simulink model "FSFB_FF_Controller"  (R2022a)
settings: Solver=VariableStepAuto  StartTime=0.0  StopTime=10.0  RelTol=1e-3
undefined symbols (not defined in the file): K1, K2
libraries: dspsigops x1
settings Model: Creator=domin  LastModifiedBy=domin

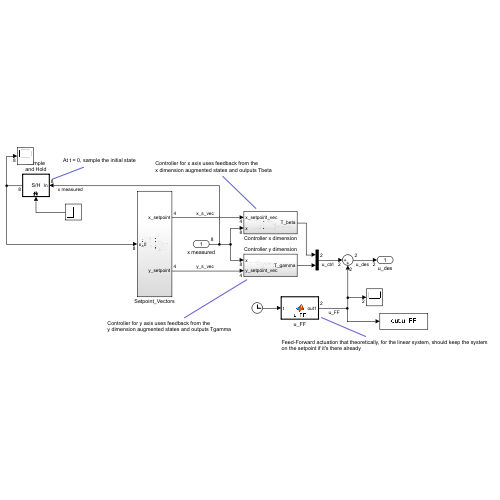
[thumbnail: Simulink's stored preview of the top-level diagram]
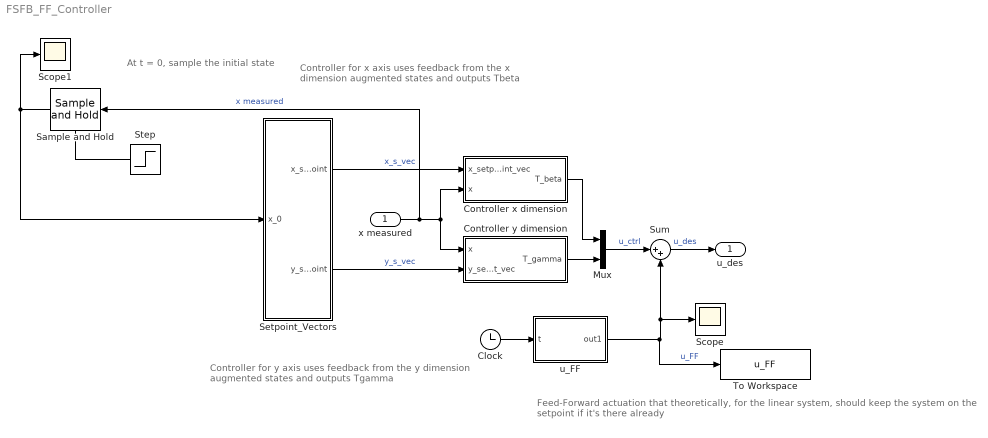
== system FSFB_FF_Controller ==
  note: Controller for x axis uses feedback from the
      | x dimension augmented states and outputs Tbeta
  note: Feed-Forward actuation that theoretically, for the linear system, should keep the system on the setpoint if it's there already
  note: Controller for y axis uses feedback from the
      | y dimension augmented states and outputs Tgamma
  note: At t = 0, sample the initial state
  x measured : Inport
  Clock : Clock
  Controller x dimension : Subsystem
  Controller y dimension : Subsystem
  Mux : Mux  Inputs=2
  Sample and Hold : dspsigops/Sample and Hold  trig=Either edge  initCond=0  latchinput=off
  Scope : Scope
  Scope1 : Scope
  Setpoint_Vectors : Subsystem
  Step : Step  Time=0  SampleTime=0
  Sum : Sum  Inputs=|++
  To Workspace : ToWorkspace  VariableName=u_FF  SampleTime=-1
  u_FF : MATLAB Function  TreatAsAtomicUnit=on
  u_des : Outport
  wires:
  Mux/1 -> Sum/1  "u_ctrl"
  u_FF/1(out1) -> To Workspace/1, Sum/2, Scope/1  "u_FF"
  Setpoint_Vectors/2(y_setpoint) -> Controller y dimension/2(y_setpoint_vec)  "y_s_vec"
  Sum/1 -> u_des/1  "u_des"
  Controller y dimension/1(T_gamma) -> Mux/2
  Clock/1 -> u_FF/1(t)
  Controller x dimension/1(T_beta) -> Mux/1
  Setpoint_Vectors/1(x_setpoint) -> Controller x dimension/1(x_setpoint_vec)  "x_s_vec"
  Sample and Hold/1 -> Setpoint_Vectors/1(x_0), Scope1/1
  Step/1 -> Sample and Hold/Trigger
  x measured/1 -> Sample and Hold/1, Controller y dimension/1(x), Controller x dimension/2(x)  "x measured"

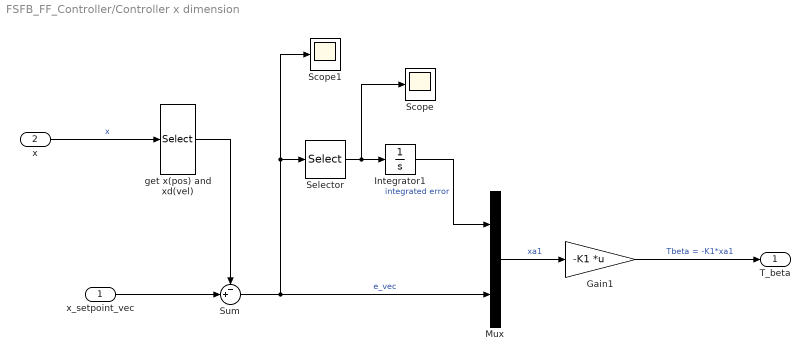
== system FSFB_FF_Controller/Controller x dimension ==
  x_setpoint_vec : Inport
  x : Inport  Port=2
  Gain1 : Gain  Gain=-K1  Multiplication=Matrix(K*u)
  Integrator1 : Integrator
  Mux : Mux  Inputs=2
  Scope : Scope
  Scope1 : Scope
  Selector : Selector  InputPortWidth=4  IndexOptions=Index vector (dialog)  Indices=[1 ]  OutputSizes=1
  Sum : Sum  Inputs=-+|
  get x(pos) and xd(vel) : Selector  InputPortWidth=8  IndexOptions=Index vector (dialog)  Indices=[1:4]  OutputSizes=1
  T_beta : Outport
  wires:
  Gain1/1 -> T_beta/1  "Tbeta = -K1*xa1"
  get x(pos) and xd(vel)/1 -> Sum/1
  Mux/1 -> Gain1/1  "xa1"
  Sum/1 -> Scope1/1, Selector/1, Mux/2  "e_vec"
  x_setpoint_vec/1 -> Sum/2
  x/1 -> get x(pos) and xd(vel)/1  "x"
  Selector/1 -> Scope/1, Integrator1/1
  Integrator1/1 -> Mux/1  "integrated error"

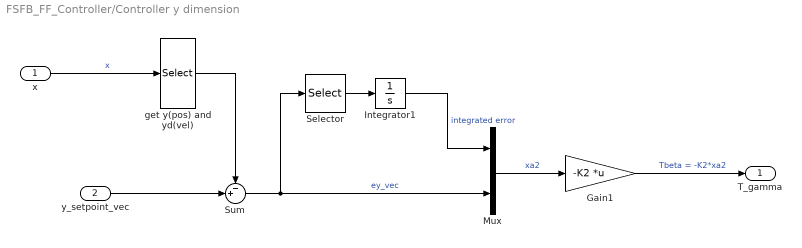
== system FSFB_FF_Controller/Controller y dimension ==
  x : Inport
  y_setpoint_vec : Inport  Port=2
  Gain1 : Gain  Gain=-K2  Multiplication=Matrix(K*u)
  Integrator1 : Integrator
  Mux : Mux  Inputs=2
  Selector : Selector  InputPortWidth=4  IndexOptions=Index vector (dialog)  Indices=[1 ]  OutputSizes=1
  Sum : Sum  Inputs=-+|
  get y(pos) and yd(vel) : Selector  InputPortWidth=8  IndexOptions=Index vector (dialog)  Indices=[5:8]  OutputSizes=1
  T_gamma : Outport
  wires:
  Integrator1/1 -> Mux/1  "integrated error"
  x/1 -> get y(pos) and yd(vel)/1  "x"
  Gain1/1 -> T_gamma/1  "Tbeta = -K2*xa2"
  get y(pos) and yd(vel)/1 -> Sum/1
  Mux/1 -> Gain1/1  "xa2"
  Selector/1 -> Integrator1/1
  Sum/1 -> Selector/1, Mux/2  "ey_vec"
  y_setpoint_vec/1 -> Sum/2

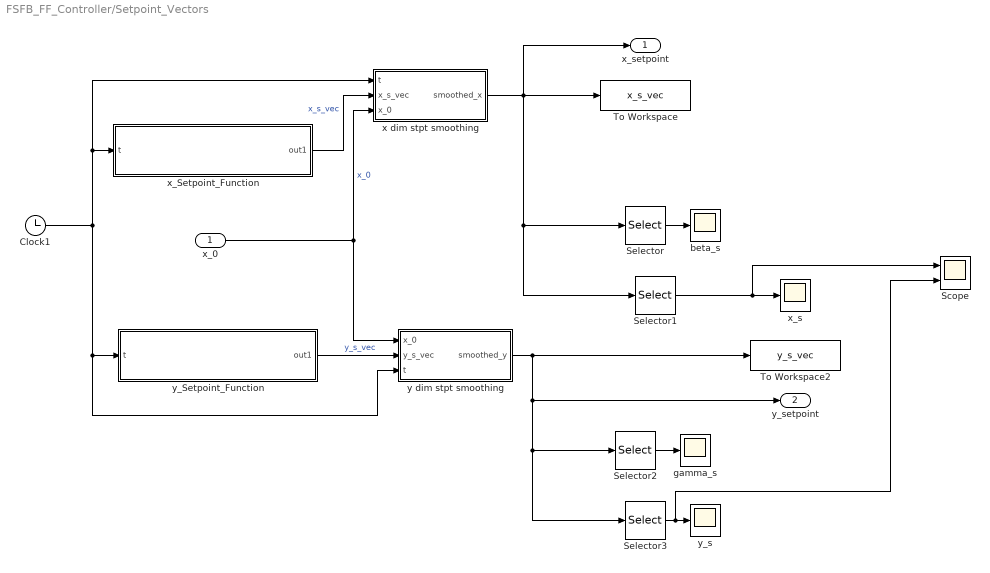
== system FSFB_FF_Controller/Setpoint_Vectors ==
  x_0 : Inport
  Clock1 : Clock
  Scope : Scope  NumInputPorts=2
  Selector : Selector  InputPortWidth=4  IndexOptions=Index vector (dialog)  Indices=[3]  OutputSizes=1
  Selector1 : Selector  InputPortWidth=4  IndexOptions=Index vector (dialog)  Indices=[1]  OutputSizes=1
  Selector2 : Selector  InputPortWidth=4  IndexOptions=Index vector (dialog)  Indices=[3]  OutputSizes=1
  Selector3 : Selector  InputPortWidth=4  IndexOptions=Index vector (dialog)  Indices=[1]  OutputSizes=1
  To Workspace : ToWorkspace  VariableName=x_s_vec  SampleTime=-1
  To Workspace2 : ToWorkspace  VariableName=y_s_vec  SampleTime=-1
  beta_s : Scope
  gamma_s : Scope
  x dim stpt smoothing : MATLAB Function  TreatAsAtomicUnit=on
  x_Setpoint_Function : MATLAB Function  TreatAsAtomicUnit=on
  x_s : Scope
  y dim stpt smoothing : MATLAB Function  TreatAsAtomicUnit=on
  y_Setpoint_Function : MATLAB Function  TreatAsAtomicUnit=on
  y_s : Scope
  x_setpoint : Outport
  y_setpoint : Outport  Port=2
  wires:
  Clock1/1 -> y_Setpoint_Function/1(t), y dim stpt smoothing/3(t), x dim stpt smoothing/1(t), x_Setpoint_Function/1(t)
  x_Setpoint_Function/1(out1) -> x dim stpt smoothing/2(x_s_vec)  "x_s_vec"
  Selector/1 -> beta_s/1
  Selector1/1 -> Scope/1, x_s/1
  Selector3/1 -> Scope/2, y_s/1
  Selector2/1 -> gamma_s/1
  y_Setpoint_Function/1(out1) -> y dim stpt smoothing/2(y_s_vec)  "y_s_vec"
  x dim stpt smoothing/1(smoothed_x) -> Selector/1, Selector1/1, To Workspace/1, x_setpoint/1
  x_0/1 -> y dim stpt smoothing/1(x_0), x dim stpt smoothing/3(x_0)  "x_0"
  y dim stpt smoothing/1(smoothed_y) -> To Workspace2/1, y_setpoint/1, Selector3/1, Selector2/1

== matlab function FSFB_FF_Controller/Setpoint_Vectors/y dim stpt smoothing ==
  data: x_0 input size=8; y_s_vec input; t input; smoothed_y output size=4; Tau parameter
function smoothed_y = fcn(x_0,y_s_vec,t, Tau)

smoothed_y = y_s_vec*(1-exp(-t/Tau)) + x_0(5:end)*exp(-t/Tau);

== matlab function FSFB_FF_Controller/Setpoint_Vectors/x_Setpoint_Function ==
  data: t input; out1 output
function out1 = x_s_vec(t)
%#codegen

%    This function was generated by the Symbolic Math Toolbox version 9.1.
%    08-Jun-2022 13:00:24

t2 = pi.^2;
t3 = t.*pi.*(2.0./5.0);
t4 = t.*pi.*(6.0./5.0);
t5 = cos(t3);
t6 = sin(t3);
t7 = t2.*1.298e+3;
t8 = t7+6.8125e+4;
t9 = t8+5.45e+5;
t10 = 1.0./t8;
t11 = 1.0./t9;
t12 = t10.*5.510882126348228e+4;
t13 = t11.*4.959793913713405e+5;
t14 = t12-5.25e+2./6.49e+2;
t15 = t13-5.25e+2./6.49e+2;
out1 = [t5.*(3.0./4.0e+1)+cos(t4).*(3.0./4.0e+1);t6.*pi.*(-3.0./1.0e+2)-pi.*sin(t4).*(9.0./1.0e+2);-t14.*(t5.*3.0-t5.^3.*4.0)+t5.*t15;t14.*(t6.*pi.*(6.0./5.0)-t5.^2.*t6.*pi.*(2.4e+1./5.0))-t6.*t15.*pi.*(2.0./5.0)];

== matlab function FSFB_FF_Controller/Setpoint_Vectors/y_Setpoint_Function ==
  data: t input; out1 output
function out1 = y_s_vec(t)
%#codegen

%    This function was generated by the Symbolic Math Toolbox version 9.1.
%    08-Jun-2022 13:00:25

t2 = pi.^2;
t3 = pi.^3;
t5 = t.*pi.*(2.0./5.0);
t6 = t.*pi.*(4.0./5.0);
t7 = t.*pi.*(6.0./5.0);
t4 = t2.^2;
t8 = cos(t5);
t9 = cos(t6);
t10 = sin(t5);
t11 = sin(t6);
t13 = t2.*8.842625e+8;
t12 = t4.*1.684804e+6;
t14 = t2.*t9.*1.298e+3;
t15 = t9.*6.13125e+5;
t16 = t12+t13+4.1769140625e+10;
t17 = t14+t15+2.725e+5;
t18 = 1.0./t16;
out1 = [t10.*(-3.0./4.0e+1)+sin(t7).*(3.0./4.0e+1);t8.*pi.*(-3.0./1.0e+2)+pi.*cos(t7).*(9.0./1.0e+2);t2.*t10.*t17.*t18.*2.1e+3;t3.*t8.*t17.*t18.*8.4e+2-t2.*t10.*t18.*(t11.*pi.*4.905e+5+t3.*t11.*1.0384e+3).*2.1e+3];

== matlab function FSFB_FF_Controller/u_FF ==
  data: out1 output size=2; t input
function out1 = u_FF(t)
%#codegen

%    This function was generated by the Symbolic Math Toolbox version 9.1.
%    08-Jun-2022 13:00:25

t2 = pi.^2;
t5 = t.*pi.*(2.0./5.0);
t6 = t.*pi.*(4.0./5.0);
t3 = t2.^2;
t4 = t2.^3;
t7 = cos(t5);
t8 = cos(t6);
t9 = sin(t5);
t10 = t2.*1.298e+3;
t13 = t2.*8.842625e+8;
t11 = t7.^3;
t12 = t3.*1.684804e+6;
t14 = t10+6.8125e+4;
t15 = t14+5.45e+5;
t16 = 1.0./t14;
t20 = t12+t13+4.1769140625e+10;
t17 = 1.0./t15;
t18 = t16.*5.510882126348228e+4;
t21 = 1.0./t20;
t19 = t17.*4.959793913713405e+5;
t22 = t18-5.25e+2./6.49e+2;
t23 = t19-5.25e+2./6.49e+2;
et1 = t2.*t9.*t21.*(-1.952921511025425e+9)-t3.*t9.*t21.*9.974023625417844e+7-t4.*t9.*t21.*1.900371767455759e+5+t8.*t9.*t21.*1.382924034667969e+10-t2.*t8.*t9.*t21.*4.101305139338456e+9-t3.*t8.*t9.*t21.*2.107185172788421e+8;
et2 = t4.*t8.*t9.*t21.*(-4.275836476775459e+5);
out1 = [t7.*(-1.6554375e-1)-cos(t.*pi.*(6.0./5.0)).*1.6554375e-1-t7.*t23.*3.412706878157143+t22.*(t7.*3.0-t11.*4.0).*3.412706878157143+t22.*(t2.*t7.*(1.2e+1./2.5e+1)-t2.*t11.*(4.8e+1./2.5e+1)+t2.*t7.*t9.^2.*(9.6e+1./2.5e+1)).*1.089342903606143e-1-t2.*t7.*t23.*1.742948645769829e-2;et1+et2];

== matlab function FSFB_FF_Controller/Setpoint_Vectors/x dim stpt smoothing ==
  data: t input; x_s_vec input size=4; smoothed_x output; Tau parameter; x_0 input
function smoothed_x = fcn(t,x_s_vec, Tau, x_0)

smoothed_x = x_s_vec*(1-exp(-t/Tau)) + x_0(1:4)*exp(-t/Tau);
